simulink library "Bit_Multiplexers_Lib"  (Simulink 8.7)
settings: Solver=ode45  StartTime=0.0  StopTime=10.0  RelTol=1e-3
settings Model: Creator=uzivatel  LastModifiedBy=Jozko Mrkvicka

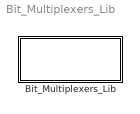
== system Bit_Multiplexers_Lib ==
  Bit_Multiplexers_Lib : Subsystem

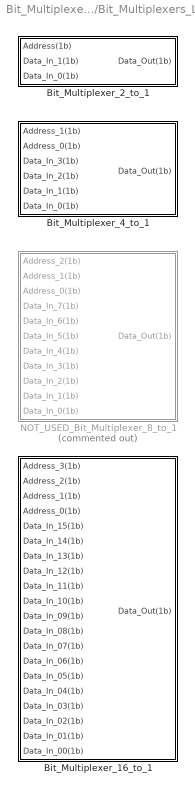
== system Bit_Multiplexers_Lib/Bit_Multiplexers_Lib ==
  Bit_Multiplexer_16_to_1 : Subsystem
  Bit_Multiplexer_2_to_1 : Subsystem
  Bit_Multiplexer_4_to_1 : Subsystem
  NOT_USED_Bit_Multiplexer_8_to_1 : Subsystem  Commented=on

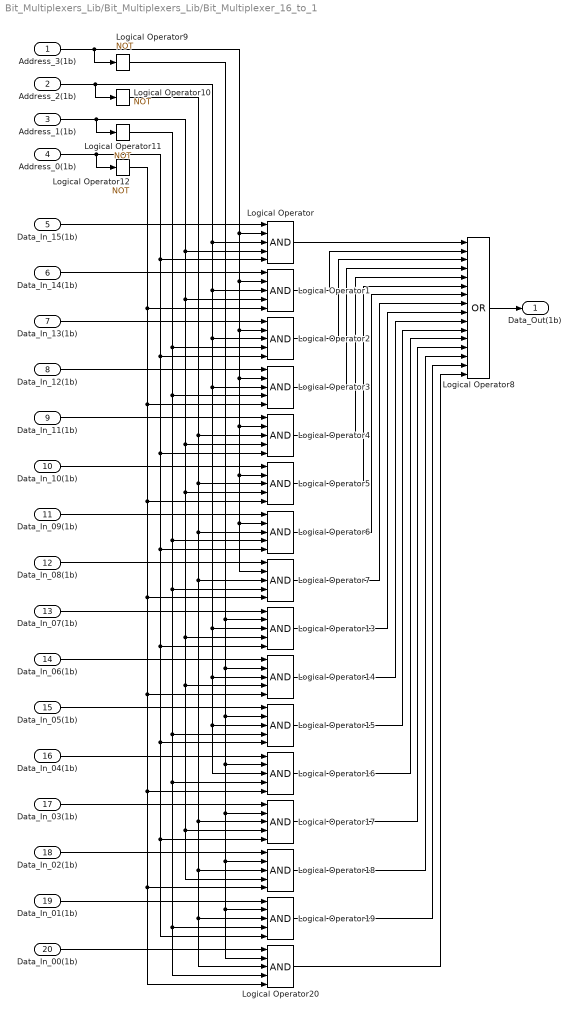
== system Bit_Multiplexers_Lib/Bit_Multiplexers_Lib/Bit_Multiplexer_16_to_1 ==
  Address_3(1b) : Inport
  Address_2(1b) : Inport  Port=2
  Address_1(1b) : Inport  Port=3
  Address_0(1b) : Inport  Port=4
  Data_In_15(1b) : Inport  Port=5
  Data_In_14(1b) : Inport  Port=6
  Data_In_13(1b) : Inport  Port=7
  Data_In_12(1b) : Inport  Port=8
  Data_In_11(1b) : Inport  Port=9
  Data_In_10(1b) : Inport  Port=10
  Data_In_09(1b) : Inport  Port=11
  Data_In_08(1b) : Inport  Port=12
  Data_In_07(1b) : Inport  Port=13
  Data_In_06(1b) : Inport  Port=14
  Data_In_05(1b) : Inport  Port=15
  Data_In_04(1b) : Inport  Port=16
  Data_In_03(1b) : Inport  Port=17
  Data_In_02(1b) : Inport  Port=18
  Data_In_01(1b) : Inport  Port=19
  Data_In_00(1b) : Inport  Port=20
  Logical Operator{,1..7,13..20} (16 alike) : Logic  Inputs=5  IconShape=distinctive  AllPortsSameDT=off  OutDataTypeStr=boolean
  Logical Operator{9..12} (4 alike) : Logic  Operator=NOT  Inputs=4  IconShape=distinctive  AllPortsSameDT=off  OutDataTypeStr=boolean
  Logical Operator8 : Logic  Operator=OR  Inputs=16  IconShape=distinctive  OutDataTypeStr=boolean
  Data_Out(1b) : Outport
  wires:
  Logical Operator12/1 -> Logical Operator20/5, Logical Operator18/5, Logical Operator16/5, Logical Operator14/5, Logical Operator7/5, Logical Operator5/5, Logical Operator3/5, Logical Operator1/5
  Address_0(1b)/1 -> Logical Operator15/5, Logical Operator17/5, Logical Operator19/5, Logical Operator13/5, Logical Operator6/5, Logical Operator4/5, Logical Operator2/5, Logical Operator/5, Logical Operator12/1
  Logical Operator11/1 -> Logical Operator20/4, Logical Operator19/4, Logical Operator16/4, Logical Operator15/4, Logical Operator7/4, Logical Operator6/4, Logical Operator3/4, Logical Operator2/4
  Address_1(1b)/1 -> Logical Operator18/4, Logical Operator17/4, Logical Operator14/4, Logical Operator13/4, Logical Operator5/4, Logical Operator4/4, Logical Operator1/4, Logical Operator/4, Logical Operator11/1
  Logical Operator10/1 -> Logical Operator20/3, Logical Operator19/3, Logical Operator18/3, Logical Operator17/3, Logical Operator7/3, Logical Operator6/3, Logical Operator5/3, Logical Operator4/3
  Address_2(1b)/1 -> Logical Operator16/3, Logical Operator15/3, Logical Operator14/3, Logical Operator13/3, Logical Operator3/3, Logical Operator2/3, Logical Operator1/3, Logical Operator/3, Logical Operator10/1
  Logical Operator9/1 -> Logical Operator20/2, Logical Operator19/2, Logical Operator18/2, Logical Operator17/2, Logical Operator16/2, Logical Operator15/2, Logical Operator14/2, Logical Operator13/2
  Address_3(1b)/1 -> Logical Operator3/2, Logical Operator4/2, Logical Operator7/2, Logical Operator6/2, Logical Operator5/2, Logical Operator2/2, Logical Operator1/2, Logical Operator/2, Logical Operator9/1
  Data_In_00(1b)/1 -> Logical Operator20/1
  Data_In_01(1b)/1 -> Logical Operator19/1
  Data_In_02(1b)/1 -> Logical Operator18/1
  Data_In_03(1b)/1 -> Logical Operator17/1
  Data_In_04(1b)/1 -> Logical Operator16/1
  Data_In_05(1b)/1 -> Logical Operator15/1
  Data_In_06(1b)/1 -> Logical Operator14/1
  Data_In_07(1b)/1 -> Logical Operator13/1
  Logical Operator20/1 -> Logical Operator8/16
  Logical Operator19/1 -> Logical Operator8/15
  Logical Operator18/1 -> Logical Operator8/14
  Logical Operator17/1 -> Logical Operator8/13
  Logical Operator16/1 -> Logical Operator8/12
  Logical Operator15/1 -> Logical Operator8/11
  Logical Operator14/1 -> Logical Operator8/10
  Logical Operator13/1 -> Logical Operator8/9
  Logical Operator8/1 -> Data_Out(1b)/1
  Data_In_15(1b)/1 -> Logical Operator/1
  Data_In_14(1b)/1 -> Logical Operator1/1
  Data_In_13(1b)/1 -> Logical Operator2/1
  Data_In_12(1b)/1 -> Logical Operator3/1
  Data_In_11(1b)/1 -> Logical Operator4/1
  Data_In_10(1b)/1 -> Logical Operator5/1
  Data_In_09(1b)/1 -> Logical Operator6/1
  Data_In_08(1b)/1 -> Logical Operator7/1
  Logical Operator7/1 -> Logical Operator8/8
  Logical Operator6/1 -> Logical Operator8/7
  Logical Operator5/1 -> Logical Operator8/6
  Logical Operator4/1 -> Logical Operator8/5
  Logical Operator3/1 -> Logical Operator8/4
  Logical Operator2/1 -> Logical Operator8/3
  Logical Operator1/1 -> Logical Operator8/2
  Logical Operator/1 -> Logical Operator8/1

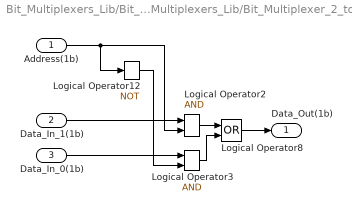
== system Bit_Multiplexers_Lib/Bit_Multiplexers_Lib/Bit_Multiplexer_2_to_1 ==
  Address(1b) : Inport
  Data_In_1(1b) : Inport  Port=2
  Data_In_0(1b) : Inport  Port=3
  Logical Operator12 : Logic  Operator=NOT  Inputs=4  IconShape=distinctive  AllPortsSameDT=off  OutDataTypeStr=boolean
  Logical Operator2 : Logic  IconShape=distinctive  AllPortsSameDT=off  OutDataTypeStr=boolean
  Logical Operator3 : Logic  IconShape=distinctive  AllPortsSameDT=off  OutDataTypeStr=boolean
  Logical Operator8 : Logic  Operator=OR  IconShape=distinctive  OutDataTypeStr=boolean
  Data_Out(1b) : Outport
  wires:
  Logical Operator12/1 -> Logical Operator3/2
  Address(1b)/1 -> Logical Operator2/2, Logical Operator12/1
  Logical Operator8/1 -> Data_Out(1b)/1
  Data_In_1(1b)/1 -> Logical Operator2/1
  Data_In_0(1b)/1 -> Logical Operator3/1
  Logical Operator3/1 -> Logical Operator8/2
  Logical Operator2/1 -> Logical Operator8/1

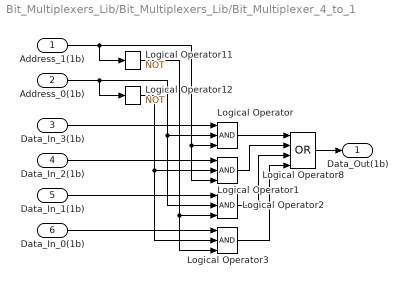
== system Bit_Multiplexers_Lib/Bit_Multiplexers_Lib/Bit_Multiplexer_4_to_1 ==
  Address_1(1b) : Inport
  Address_0(1b) : Inport  Port=2
  Data_In_3(1b) : Inport  Port=3
  Data_In_2(1b) : Inport  Port=4
  Data_In_1(1b) : Inport  Port=5
  Data_In_0(1b) : Inport  Port=6
  Logical Operator{,1..3} (4 alike) : Logic  Inputs=3  IconShape=distinctive  AllPortsSameDT=off  OutDataTypeStr=boolean
  Logical Operator11 : Logic  Operator=NOT  Inputs=4  IconShape=distinctive  AllPortsSameDT=off  OutDataTypeStr=boolean
  Logical Operator12 : Logic  Operator=NOT  Inputs=4  IconShape=distinctive  AllPortsSameDT=off  OutDataTypeStr=boolean
  Logical Operator8 : Logic  Operator=OR  Inputs=4  IconShape=distinctive  OutDataTypeStr=boolean
  Data_Out(1b) : Outport
  wires:
  Logical Operator12/1 -> Logical Operator3/2, Logical Operator1/2
  Address_0(1b)/1 -> Logical Operator2/2, Logical Operator/2, Logical Operator12/1
  Logical Operator11/1 -> Logical Operator3/3, Logical Operator2/3
  Address_1(1b)/1 -> Logical Operator1/3, Logical Operator/3, Logical Operator11/1
  Logical Operator8/1 -> Data_Out(1b)/1
  Data_In_3(1b)/1 -> Logical Operator/1
  Data_In_2(1b)/1 -> Logical Operator1/1
  Data_In_1(1b)/1 -> Logical Operator2/1
  Data_In_0(1b)/1 -> Logical Operator3/1
  Logical Operator3/1 -> Logical Operator8/4
  Logical Operator2/1 -> Logical Operator8/3
  Logical Operator1/1 -> Logical Operator8/2
  Logical Operator/1 -> Logical Operator8/1

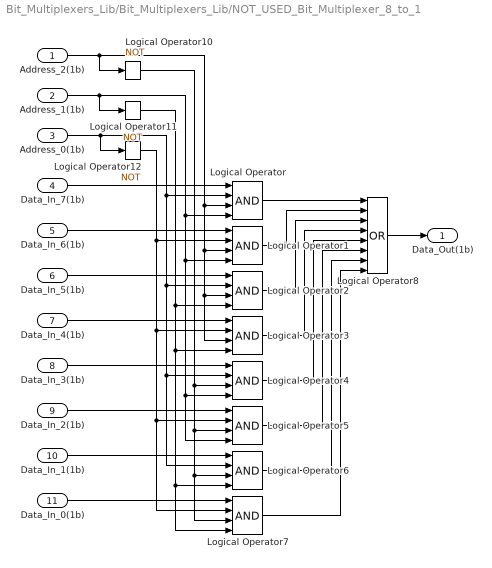
== system Bit_Multiplexers_Lib/Bit_Multiplexers_Lib/NOT_USED_Bit_Multiplexer_8_to_1 ==
  Address_2(1b) : Inport
  Address_1(1b) : Inport  Port=2
  Address_0(1b) : Inport  Port=3
  Data_In_7(1b) : Inport  Port=4
  Data_In_6(1b) : Inport  Port=5
  Data_In_5(1b) : Inport  Port=6
  Data_In_4(1b) : Inport  Port=7
  Data_In_3(1b) : Inport  Port=8
  Data_In_2(1b) : Inport  Port=9
  Data_In_1(1b) : Inport  Port=10
  Data_In_0(1b) : Inport  Port=11
  Logical Operator{,1..7} (8 alike) : Logic  Inputs=4  IconShape=distinctive  AllPortsSameDT=off  OutDataTypeStr=boolean
  Logical Operator10 : Logic  Operator=NOT  Inputs=4  IconShape=distinctive  AllPortsSameDT=off  OutDataTypeStr=boolean
  Logical Operator11 : Logic  Operator=NOT  Inputs=4  IconShape=distinctive  AllPortsSameDT=off  OutDataTypeStr=boolean
  Logical Operator12 : Logic  Operator=NOT  Inputs=4  IconShape=distinctive  AllPortsSameDT=off  OutDataTypeStr=boolean
  Logical Operator8 : Logic  Operator=OR  Inputs=8  IconShape=distinctive  OutDataTypeStr=boolean
  Data_Out(1b) : Outport
  wires:
  Logical Operator12/1 -> Logical Operator7/2, Logical Operator5/2, Logical Operator3/2, Logical Operator1/2
  Address_0(1b)/1 -> Logical Operator12/1, Logical Operator6/2, Logical Operator4/2, Logical Operator2/2, Logical Operator/2
  Logical Operator11/1 -> Logical Operator7/4, Logical Operator6/4, Logical Operator3/4, Logical Operator2/4
  Address_1(1b)/1 -> Logical Operator11/1, Logical Operator5/4, Logical Operator4/4, Logical Operator1/4, Logical Operator/4
  Logical Operator10/1 -> Logical Operator7/3, Logical Operator6/3, Logical Operator5/3, Logical Operator4/3
  Address_2(1b)/1 -> Logical Operator3/3, Logical Operator2/3, Logical Operator1/3, Logical Operator/3, Logical Operator10/1
  Logical Operator8/1 -> Data_Out(1b)/1
  Data_In_7(1b)/1 -> Logical Operator/1
  Data_In_6(1b)/1 -> Logical Operator1/1
  Data_In_5(1b)/1 -> Logical Operator2/1
  Data_In_4(1b)/1 -> Logical Operator3/1
  Data_In_3(1b)/1 -> Logical Operator4/1
  Data_In_2(1b)/1 -> Logical Operator5/1
  Data_In_1(1b)/1 -> Logical Operator6/1
  Data_In_0(1b)/1 -> Logical Operator7/1
  Logical Operator7/1 -> Logical Operator8/8
  Logical Operator6/1 -> Logical Operator8/7
  Logical Operator5/1 -> Logical Operator8/6
  Logical Operator4/1 -> Logical Operator8/5
  Logical Operator3/1 -> Logical Operator8/4
  Logical Operator2/1 -> Logical Operator8/3
  Logical Operator1/1 -> Logical Operator8/2
  Logical Operator/1 -> Logical Operator8/1
